simulink model "saturation"  (R2023b)
settings: Solver=VariableStepAuto  StartTime=0.0  StopTime=10.0  RelTol=1e-3
settings Model: Creator=pratikmandi  LastModifiedBy=pratikmandi

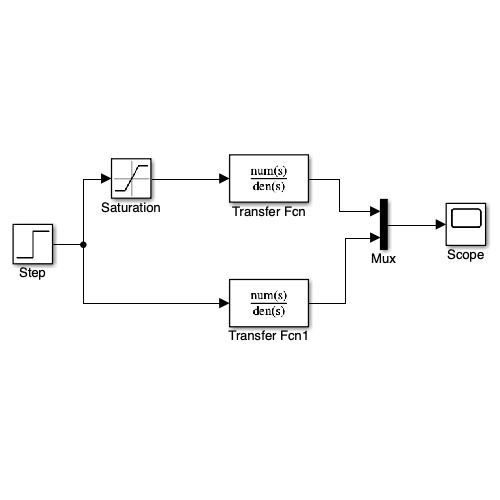
[thumbnail: Simulink's stored preview of the top-level diagram]
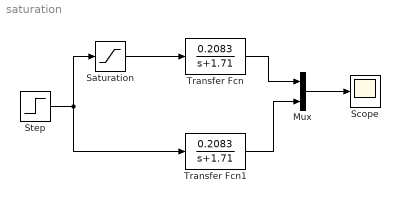
== system saturation ==
  Mux : Mux  Inputs=2
  Saturation : Saturate
  Scope : Scope
  Step : Step  SampleTime=0
  Transfer Fcn : TransferFcn  Numerator=[0.2083]  Denominator=[1 1.71]
  Transfer Fcn1 : TransferFcn  Numerator=[0.2083]  Denominator=[1 1.71]
  wires:
  Saturation/1 -> Transfer Fcn/1
  Step/1 -> Transfer Fcn1/1, Saturation/1
  Transfer Fcn/1 -> Mux/1
  Transfer Fcn1/1 -> Mux/2
  Mux/1 -> Scope/1
